simulink model "Custom_SP"  (R2020b)
settings: Solver=ode45  StartTime=0.0  StopTime=TimeScale  RelTol=1e-3
model workspace (MATLAB code in the model file):
  | %% PARAMETERS FOR CUSTOM_SP
  | %%%%%%%%%%%%%%%%%%%%% DENSITY %%%%%%%%%%%%%%%%%%%%%%%
  | al = 2.07; % g/cm^3
  | steel = 7.833; %g/cm^3
  | 
  | %%%%%%%%%%%%%%%%%%%%% BASE COORDINATES %%%%%%%%%%%%%%%%%%%%%%%
  | % Outside coordinates
  | out_base_right = [-335 -170.32; -315 -204.96;
  |     -315 -295.6; -98.49 -420.6; -20 -375.28;
  |     20 -375.28; 315 -204.96; 335 -170.32; 413.49 -125];
  | out_base_left = [413.49 125; 335 170.32;
  |     315 204.96; 20 375.28; -20 375.28;
  |     -98.49 420.6; -315 295.6; -315 204.96; -335 170.32;
  |     -335 -170.32];
  | out_base = [out_base_right; out_base_left];
  | 
  | % Inside coordinates
  | in_base = [-230 -246.52; -230 246.52; -98.49 322.45; 328.49 75.93;
  |     328.49 -75.93; -98.49 -322.45; -230 -246.52];
  | 
  | tot_base = [out_base; in_base];
  | 
  | %%%%%%%%%%%%%%%%%%%%%%% PLATE POSE ON BASE %%%%%%%%%%%%%%%%%%%%%%%%%%%
  | % PLATE POSITION ON BASE
  | plate_1 = [-272.22 -252.09 0];
  | plate_2 = [-82.21 -361.79 0];
  | plate_3 = [354.42 -109.71 0];
  | plate_4 = [354.42 109.71 0];
  | plate_5 = [-82.21 361.79 0];
  | plate_6 = [-272.22  252.09 0];
  | 
  | % ANGLE FOR JOINT ON BASE
  | plate_angle_1 = 0 + pi/2;
  | plate_angle_2 = 2*pi/3 + pi/2;
  | plate_angle_3 = 2*pi/3 + pi/2;
  | plate_angle_4 = 4*pi/3 + pi/2;
  | plate_angle_5 = 4*pi/3 + pi/2;
  | plate_angle_6 = 0 + pi/2;
  | 
  | %%%%%%%%%%%%%%%%%%%%%%%% FLANGE COORDINATES %%%%%%%%%%%%%%%%%%%%%%%%%%%%
  | flange_body = [ -20 22.5; -20 -22.5; 13.6488 -9.3106];
  | 
  | C = linspace(-68.6, 68.6, 21)';
  | C = deg2rad(C);
  | flange_round = [10+10*cos(C) 10*sin(C)];
  | 
  | C = linspace(3*pi/2, -pi/2, 100)';
  | flange_hole = [10+6*cos(C) 6*sin(C)];
  | 
  | flange = [flange_round; flange_body; flange_hole];
  | 
  | %plot(flange(:,1),flange(:,2), 'Color', [0.6 0.6 0.6], 'Marker', '.',...
  | %'MarkerSize', 9, 'MarkerEdgeColor', [1 0 0]);
  | 
  | %%%%%%%%%%%%%%%%%%%%%%%%%%%%% LID %%%%%%%%%%%%%%%%%%%%%%%%%%%%%%
  | % LID COORDINATES
  | C = linspace(-150 , -70, 9)';
  | C = deg2rad(C);
  | lid_round1 = [-171.37+10*cos(C) -103.18+10*sin(C)];
  | 
  | C = linspace(110, 60, 9)';
  | C = deg2rad(C);
  | lid_round2 = [-118.05+10*cos(C) -105.05+10*sin(C)];
  | 
  | C = linspace(60, 10, 9)';
  | C = deg2rad(C);
  | lid_round3 = [-117.46+10*cos(C) -105.39+10*sin(C)];
  | 
  | C = linspace(110, 60, 9)';
  | C = deg2rad(C);
  | lid_round4 = [-32.54+10*cos(C) -154.42+10*sin(C)];
  | 
  | C = linspace(60, 10, 9)';
  | C = deg2rad(C);
  | lid_round5 = [-31.95+10*cos(C) -154.76+10*sin(C)];
  | 
  | C = linspace(-90-80, -90, 9)';
  | C = deg2rad(C);
  | lid_round6 = [-3.67+10*cos(C) -200+10*sin(C)];
  | 
  | C = linspace(-30, 50, 9)';
  | C = deg2rad(C);
  | lid_round7 = [175.04+10*cos(C) -96.82+10*sin(C)];
  | 
  | C = linspace(-140, -90, 9)';
  | C = deg2rad(C);
  | lid_round8 = [150+10*sin(C) -49.71+10*cos(C)];
  | 
  | C = linspace(-90, -40, 9)';
  | C = deg2rad(C);
  | lid_round9 = [150+10*sin(C) -49.03+10*cos(C)];
  | 
  | C = linspace(-140, -90, 9)';
  | C = deg2rad(C);
  | lid_round10 = [150+10*sin(C) 49.03+10*cos(C)];
  | 
  | C = linspace(-90, -40, 9)';
  | C = deg2rad(C);
  | lid_round11 = [150+10*sin(C) 49.71+10*cos(C)];
  | 
  | C = linspace(-50, 30, 9)';
  | C = deg2rad(C);
  | lid_round12 = [175.04+10*cos(C) 96.82+10*sin(C)];
  | 
  | C = linspace(90, 90+80, 9)';
  | C = deg2rad(C);
  | lid_round13 = [-3.67+10*cos(C) 200+10*sin(C)];
  | 
  | C = linspace(-10, -60, 9)';
  | C = deg2rad(C);
  | lid_round14 = [-31.95+10*cos(C) 154.76+10*sin(C)];
  | 
  | C = linspace(-60, -110, 9)';
  | C = deg2rad(C);
  | lid_round15 = [-32.54+10*cos(C) 154.42+10*sin(C)];
  | 
  | C = linspace(-10, -60, 9)';
  | C = deg2rad(C);
  | lid_round16 = [-117.46+10*cos(C) 105.39+10*sin(C)];
  | 
  | C = linspace(-60, -110, 9)';
  | C = deg2rad(C);
  | lid_round17 = [-118.05+10*cos(C) 105.05+10*sin(C)];
  | 
  | C = linspace(70 , 150, 9)';
  | C = deg2rad(C);
  | lid_round18 = [-171.37+10*cos(C) 103.18+10*sin(C)];
  | 
  | lid = [-200 -73.59; lid_round1; lid_round2;
  |     lid_round3;
  |     -100.49 -144.05; -74.51 -159.05; lid_round4;
  |     lid_round5; lid_round6; 36.27 -210; 163.73 -136.41;
  |     lid_round7; lid_round8; lid_round9; 175 -15; 175 15;
  |     lid_round10; lid_round11; lid_round12; 163.73 136.41;
  |     36.27 210; lid_round13; lid_round14; lid_round15;
  |     -74.51 159.05; -100.49 144.05; lid_round16;
  |     lid_round17; lid_round18; -200 73.59];
  | 
  | lid = [-200 -73.59; lid_round1; lid_round2; lid_round3;
  |     -100.49 -144.05; -74.51 -159.05;
  |     lid_round4; lid_round5; lid_round6;
  |     36.27 -210; 163.73 -136.41;
  |     lid_round7; lid_round8; lid_round9;
  |     175 -15; 175 15;
  |     lid_round10; lid_round11; lid_round12;
  |     163.73 136.41; 36.27 210;
  |     lid_round13; lid_round14; lid_round15;
  |     -74.51 159.05; -100.49 144.05;
  |     lid_round16; lid_round17; lid_round18; -200 73.59];
  | 
  | % LID CONNECTOR
  | C = linspace(-150 , -50, 15)';
  | C = deg2rad(C);
  | lid_connector_round1 = [2.15+10*cos(C) -79.37+10*sin(C)];
  | 
  | C = linspace(-50 , 0, 15)';
  | C = deg2rad(C);
  | lid_connector_round2 = [37.5+10*cos(C) -49.71+10*sin(C)];
  | 
  | C = linspace(0 , 50, 15)';
  | C = deg2rad(C);
  | lid_connector_round3 = [37.5+10*cos(C) -49.03+10*sin(C)];
  | 
  | C = linspace(-50, 0, 15)';
  | C = deg2rad(C);
  | lid_connector_round4 = [37.5+10*cos(C) 49.03+10*sin(C)];
  | 
  | C = linspace(0, 50, 15)';
  | C = deg2rad(C);
  | lid_connector_round5 = [37.5+10*cos(C) 49.71+10*sin(C)];
  | 
  | C = linspace(50 , 150, 15)';
  | C = deg2rad(C);
  | lid_connector_round6 = [2.15+10*cos(C) 79.37+10*sin(C)];
  | 
  | lid_connector = [-12.5 -74; lid_connector_round1;
  |     lid_connector_round2; lid_connector_round3; 12.5 -15;
  |     12.5 15; lid_connector_round4; lid_connector_round5;
  |     lid_connector_round6; -12.5 74];
  | 
  | %%%%%%%%%%%%%%%%%%%%%%%%% BALL JOINT %%%%%%%%%%%%%%%%%%%%%%%%%%%
  | % BALL JOINTS
  | C = linspace(138.59, 41.41, 50)';
  | C = deg2rad(C);
  | ball_round = [10*sin(C) 10*cos(C)];
  | 
  | ball_joint = [6 -7.5; ball_round; 6 7.5];
  | 
  | % BALL CONNECTOR
  | C = linspace(-109.47, -70.53, 49)';
  | C = deg2rad(C);
  | ball_round_out = [-16*sin(C) 16*cos(C)];
  | 
  | C = linspace(-57.75, -122.25, 49)';
  | C = deg2rad(C);
  | ball_round_in = [-10*sin(C) 10*cos(C)];
  | 
  | ball_connector = [ball_round_out; ball_round_in];
  | 
  | %%%%%%%%%%%%%%%%%%%%%%%%%% MOTOR %%%%%%%%%%%%%%%%%%%%%%%%%%%
  | % KNOB UNDER MOTOR
  | C = linspace(-90+25.84, -90+64.16, 50)';
  | C = deg2rad(C);
  | knob_under_round1 = [7.5*sin(C) -7.5*cos(C)];
  | 
  | C = linspace( -64.16, -25.84, 50)';
  | C = deg2rad(C);
  | knob_under_round2 = [7.5*cos(C) 7.5*sin(C)];
  | 
  | C = linspace( 25.84, 64.16, 50)';
  | C = deg2rad(C);
  | knob_under_round3 = [7.5*cos(C) 7.5*sin(C)];
  | 
  | C = linspace( 64.16, 25.84, 50)';
  | C = deg2rad(C);
  | knob_under_round4 = [-7.5*cos(C) 7.5*sin(C)];
  | 
  | knob_under = [knob_under_round1; knob_under_round2;
  |     knob_under_round3; knob_under_round4];
  | 
  | % MOTOR UNDER
  | C = linspace(-90, -49, 10)';
  | C = deg2rad(C);
  | knob_under_round1 = [-(19+17)+5.5*sin(C) -11.13-5.5*cos(C)];
  | 
  | C = linspace(-49, 0, 10)';
  | C = deg2rad(C);
  | knob_under_round2 = [-(17+14.77)+5.5*sin(C) -16-5.5*cos(C)];
  | 
  | C = linspace(0, 180, 49)';
  | C = deg2rad(C);
  | knob_under_round3 = [20+21.5*sin(C) -21.5*cos(C)];
  | 
  | C = linspace(180, 180+49, 10)';
  | C = deg2rad(C);
  | knob_under_round4 = [-(17+14.77)+5.5*sin(C) 16-5.5*cos(C)];
  | 
  | C = linspace(270-49, 270, 10)';
  | C = deg2rad(C);
  | knob_under_round5 = [-(19+17)+5.5*sin(C) 11.13-5.5*cos(C)];
  | 
  | motor_under = [knob_under_round1; knob_under_round2;
  |     knob_under_round3; knob_under_round4; knob_under_round5];
  | 
  | % MOTOR LINEAR
  | C = linspace(-180, -101.99, 10)';
  | C = deg2rad(C);
  | motor_top_round1 = [-15.28+3*cos(C) -8.62+3*sin(C)];
  | 
  | C = linspace(-101.99, 101.99, 49)';
  | C = deg2rad(C);
  | motor_top_round2 = [3.12+15.25*cos(C) 15.25*sin(C)];
  | 
  | C = linspace(101.99, 180, 10)';
  | C = deg2rad(C);
  | motor_top_round3 = [-15.28+3*cos(C) 8.62+3*sin(C)];
  | 
  | C = linspace(180, -180, 50)';
  | C = deg2rad(C);
  | motor_top_hole = [3.12+10.1*cos(C) 10.1*sin(C)];
  | 
  | motor_linear = [motor_top_round1; motor_top_round2; motor_top_round3;
  |     -15.28-3 -8.62; motor_top_hole];
  | 
  | %%%%%%%%%%%%%%%%%%%%% MALE %%%%%%%%%%%%%%%%%%%%%%%%%%%
  | male = [15.1 -16; 15.1 16; 10.1 16;
  |     10.1 -11; 6 -11; 6 -16];
  | 
  | %%%%%%%%%%%%%%%%%%%%% FEMALE %%%%%%%%%%%%%%%%%%%%%%%%%
  | female = [15 -19; 15 19; 9.5 19; 9.5 1;
  |     5.055 1; 5.055 -19];
  | 
  | %%%%%%%%%%%%%%%%%%%%% STRAIN GAUGE %%%%%%%%%%%%%%%%%%%%%%
  | strain_gauge = [-38.1 -25.4; -22.4 -25.4; -22.4 11.6;
  |     -13.9 11.6; -13.9 -25.4; 38.1 -25.4; 38.1 25.4;
  |     22.4 25.4; 22.4 -11.6; 13.9 -11.6;
  |     13.9 25.4; -38.1 25.4];
  | 
  | %%%%%%%%%%%%%%%%%%%%% M12 STUFF %%%%%%%%%%%%%%%%%%%%%%%%%%%
  | % M12 BOLT
  | m12_bolt = [0 -18.5; 6 -18.5; 6 11.5; 10.1 11.5; 10.1 18.5; 0 18.5];
  | 
  | % M12 NUT
  | C = linspace(3*pi, pi, 50)';
  | m12_hole = [6*cos(C) 6*sin(C)];
  | m12_nut = [-21.2/2 0; -5.48 -9.5; 5.48 -9.5; 21.2/2 0; 5.48 9.5; -5.48 9.5; -21.2/2 0; m12_hole];
  | 
  | % M12 WASHER
  | m12_washer = [6 -1; 23.5/2 -1; 23.5/2 1; 6 1];
  | 
  | %%%%%%%%%%%%%%%%%%%%%% PLATFORM COORDINATES %%%%%%%%%%%%%%%%%%%%%%%%%%%
  | % Outside coordinates
  | out_platform = [36.27 -210; 163.73 -136.41;
  |     200 -73.59; 200 73.59; 163.73 136.41;
  |     36.27 210; -36.27 210; -163.73 136.41;
  |     -200 73.59; -200 -73.54; -163.73 -136.41; -36.27 -210;
  |     36.27 -210];
  | C = linspace(3*pi/2, -pi/2, 100)';
  | platform_hole = [140*cos(C) 140*sin(C)];
  | platform = [out_platform; platform_hole];
  | 
  | %%%%%%%%%%%%%%%%%%%% STUMP %%%%%%%%%%%%%%%%%%%%%%%
  | C = linspace(-pi/2, -deg2rad(12.47), 100)';
  | stump_round = [70*cos(C) -100+70*sin(C)];
  | stump = [stump_round; 100 170; 0 170];
  | 
  | %% POSITION OF BASE JOINT AND PLATFORM JOINT FOR INVERSE KINEMATICS
  | % BASE JOINT POSITION
  | plate_1;
  | plate_2;
  | plate_3;
  | plate_4;
  | plate_5;
  | plate_6;
  | 
  | zb = 35+5;
  | B = [plate_1 zb; plate_2 zb; plate_3 zb; plate_4 zb; plate_5 zb; plate_6 zb]';
  | 
  | 
  | % JOINT POSITION ON PLATFORM
  | Rot = [cos(deg2rad(120)) -sin(deg2rad(120)); sin(deg2rad(120)) cos(deg2rad(120))];
  | platform_joint_1 = [-200.54 -48.83]';
  | platform_joint_6 = [-200.54 48.83]';
  | platform_joint_2 = Rot*platform_joint_6;
  | platform_joint_3 = Rot*platform_joint_1;
  | platform_joint_4 = Rot*platform_joint_2;
  | platform_joint_5 = Rot*platform_joint_3;
  | 
  | % LEG LENGHT AT HOME POSITION
  | %ball_joint_bottom_length = 13.75; %mm
  | %nut_washer = 10 + 2 + 7.75; %mm
  | %female_length = 38 + 2; %mm
  | %motor_length = 58.5 + 163.5; %mm
  | %extender_length = 20 + 50; %mm
  | %male_bolt_nut = 5 + 7 + 25; %mm
  | %strain_gauge_length = 38.1*2; %mm
  | %nut = 10 + 7.75; %mm
  | %ball_joint_top_length = 13.75; %mm
  | 
  | %leg_initial_length = ball_joint_bottom_length + nut_washer + female_length + motor_length + extender_length + male_bolt_nut + strain_gauge_length + nut + ball_joint_top_length;
  | 
  | %leg_initial_length = 510.2061739;
  | 
  | %height_home = sqrt(leg_initial_length^2 - (plate_1(1)-platform_joint_1(1))^2 - (plate_1(2)-platform_joint_1(2))^2) + zb;
  | height_home = 503.318 + 2.5;
  | P = [platform_joint_1' height_home; platform_joint_2' height_home; platform_joint_3' height_home; platform_joint_4' height_home; platform_joint_5' height_home; platform_joint_6' height_home]';
values from neighbouring files (symbols this model uses):
  LegSpring = 50000    [SP_parameters.m]
undefined symbols (not defined in the file or in its folder): X, Y, Z
libraries: nesl_utility x13, Custom_SP_lib x8, sm_lib x7, simulink x6
settings Model: Creator=ellen  LastModifiedBy=axelzedigh

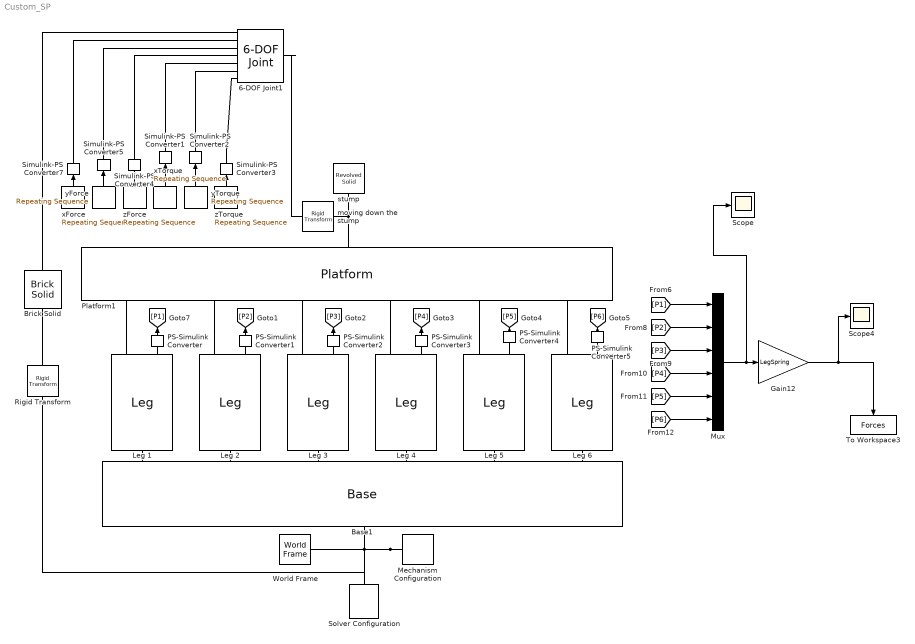
== system Custom_SP ==
  6-DOF Joint1 : sm_lib/Joints/6-DOF Joint  JointMode=Normal  SenseConstraintForce=off  SenseConstraintForceX=off  SenseConstraintForceY=off  SenseConstraintForceZ=off  SenseConstraintTorque=off  SenseConstraintTorqueX=off  SenseConstraintTorqueY=off  SenseConstraintTorqueZ=off  SenseTotalForce=off  SenseTotalForceX=off  SenseTotalForceY=off  SenseTotalForceZ=off  SenseTotalTorque=off  SenseTotalTorqueX=off  SenseTotalTorqueY=off  SenseTotalTorqueZ=off  CompositeWrenchDir=FollowerOnBase  CompositeWrenchFrame=BaseFrame  PxEquilibriumPosition=0  PxEquilibriumPositionUnits=m  PxSpringStiffness=0  PxSpringStiffnessUnits=N/m  PxDampingCoefficient=0  PxDampingCoefficientUnits=N/(m/s)  PxTorqueActuationMode=InputTorque  PxMotionActuationMode=ComputedMotion  PxSensePosition=off  PxSenseVelocity=off  PxSenseAcceleration=off  PxSenseTorqueForce=off  PxSenseLowerLimitTorqueForce=off  PxSenseUpperLimitTorqueForce=off  PxLowerLimitSpecify=off  PxLowerLimitBound=-1  PxLowerLimitBoundUnits=m  PxLowerLimitStiffness=1e6  PxLowerLimitStiffnessUnits=N/m  PxLowerLimitDamping=1e3  PxLowerLimitDampingUnits=N/(m/s)  PxLowerLimitTransitionRegionWidth=1e-4  PxLowerLimitTransitionRegionWidthUnits=m  PxUpperLimitSpecify=off  PxUpperLimitBound=1  PxUpperLimitBoundUnits=m  PxUpperLimitStiffness=1e6  PxUpperLimitStiffnessUnits=N/m  PxUpperLimitDamping=1e3  PxUpperLimitDampingUnits=N/(m/s)  PxUpperLimitTransitionRegionWidth=1e-4  PxUpperLimitTransitionRegionWidthUnits=m  PxPositionTargetSpecify=off  PxPositionTargetPriority=High  PxPositionTargetValue=0  PxPositionTargetValueUnits=m  PxVelocityTargetSpecify=off  PxVelocityTargetPriority=High  PxVelocityTargetValue=0  PxVelocityTargetValueUnits=m/s  PyEquilibriumPosition=0  PyEquilibriumPositionUnits=m  PySpringStiffness=0  PySpringStiffnessUnits=N/m  PyDampingCoefficient=0  PyDampingCoefficientUnits=N/(m/s)  PyTorqueActuationMode=InputTorque  PyMotionActuationMode=ComputedMotion  PySensePosition=off  PySenseVelocity=off  PySenseAcceleration=off  PySenseTorqueForce=off  PySenseLowerLimitTorqueForce=off  PySenseUpperLimitTorqueForce=off  PyLowerLimitSpecify=off  PyLowerLimitBound=-1  PyLowerLimitBoundUnits=m  PyLowerLimitStiffness=1e6  PyLowerLimitStiffnessUnits=N/m  PyLowerLimitDamping=1e3  PyLowerLimitDampingUnits=N/(m/s)  PyLowerLimitTransitionRegionWidth=1e-4  PyLowerLimitTransitionRegionWidthUnits=m  PyUpperLimitSpecify=off  PyUpperLimitBound=1  PyUpperLimitBoundUnits=m  PyUpperLimitStiffness=1e6  PyUpperLimitStiffnessUnits=N/m  PyUpperLimitDamping=1e3  PyUpperLimitDampingUnits=N/(m/s)  PyUpperLimitTransitionRegionWidth=1e-4  PyUpperLimitTransitionRegionWidthUnits=m  PyPositionTargetSpecify=off  PyPositionTargetPriority=High  PyPositionTargetValue=0  PyPositionTargetValueUnits=m  PyVelocityTargetSpecify=off  PyVelocityTargetPriority=High  PyVelocityTargetValue=0  PyVelocityTargetValueUnits=m/s  PzEquilibriumPosition=0  PzEquilibriumPositionUnits=m  PzSpringStiffness=0  PzSpringStiffnessUnits=N/m  PzDampingCoefficient=0  PzDampingCoefficientUnits=N/(m/s)  PzTorqueActuationMode=InputTorque  PzMotionActuationMode=ComputedMotion  PzSensePosition=off  PzSenseVelocity=off  PzSenseAcceleration=off  PzSenseTorqueForce=off  PzSenseLowerLimitTorqueForce=off  PzSenseUpperLimitTorqueForce=off  PzLowerLimitSpecify=off  PzLowerLimitBound=-1  PzLowerLimitBoundUnits=m  PzLowerLimitStiffness=1e6  PzLowerLimitStiffnessUnits=N/m  PzLowerLimitDamping=1e3  PzLowerLimitDampingUnits=N/(m/s)  PzLowerLimitTransitionRegionWidth=1e-4  PzLowerLimitTransitionRegionWidthUnits=m  PzUpperLimitSpecify=off  PzUpperLimitBound=1  PzUpperLimitBoundUnits=m  PzUpperLimitStiffness=1e6  PzUpperLimitStiffnessUnits=N/m  PzUpperLimitDamping=1e3  PzUpperLimitDampingUnits=N/(m/s)  PzUpperLimitTransitionRegionWidth=1e-4  PzUpperLimitTransitionRegionWidthUnits=m  PzPositionTargetSpecify=off  PzPositionTargetPriority=High  PzPositionTargetValue=0  PzPositionTargetValueUnits=m  PzVelocityTargetSpecify=off  PzVelocityTargetPriority=High  PzVelocityTargetValue=0  PzVelocityTargetValueUnits=m/s  SphDefPosRotationMethod=None  SphDefPosRotationAngleUnits=deg  SphDefPosRotationStandardAxis=+Z  SphDefPosRotationAngle=0.0  SphDefPosRotationArbitraryAxis=[0 0 1]  SphDefPosFollAlignAxisA=+X  SphDefPosBaseAlignAxisA=+Y  SphDefPosFollAlignAxisB=+Y  SphDefPosBaseAlignAxisB=+Z  SphDefPosRotationSequenceAxes=FollowerAxes  SphDefPosRotationSequence=XYX  SphDefPosRotationSequenceAngles=[0 0 0]  SphDefPosRotationSequenceAnglesUnits=deg  SphDefPosRotationMatrix=[1 0 0; 0 1 0; 0 0 1]  SphEqPosRotationMethod=None  SphEqPosRotationAngleUnits=deg  SphEqPosRotationStandardAxis=+Z  SphEqPosRotationAngle=0.0  SphEqPosRotationArbitraryAxis=[0 0 1]  SphEqPosFollAlignAxisA=+X  SphEqPosBaseAlignAxisA=+Y  SphEqPosFollAlignAxisB=+Y  SphEqPosBaseAlignAxisB=+Z  SphEqPosRotationSequenceAxes=FollowerAxes  SphEqPosRotationSequence=XYX  SphEqPosRotationSequenceAngles=[0 0 0]  SphEqPosRotationSequenceAnglesUnits=deg  SphEqPosRotationMatrix=[1 0 0; 0 1 0; 0 0 1]  SphSpringStiffness=0  SphSpringStiffnessUnits=N*m/deg  SphDampingCoefficient=0  SphDampingCoefficientUnits=N*m/(deg/s)  SphActuateTorqueX=on  SphActuateTorqueY=on  SphActuateTorqueZ=on  SphActuateTorque=off  SphTorqueActuationMode=InputTorque  SphMotionActuationMode=ComputedMotion  SphActuationFrame=BaseFrame  SphSensePosition=off  SphSenseVelocityX=off  SphSenseVelocityY=off  SphSenseVelocityZ=off  SphSenseVelocity=off  SphSenseAccelerationX=off  SphSenseAccelerationY=off  SphSenseAccelerationZ=off  SphSenseAcceleration=off  SphSenseTorqueX=off  SphSenseTorqueY=off  SphSenseTorqueZ=off  SphSenseTorqueForce=off  SphSenseLowerLimitTorqueMag=off  SphSenseUpperLimitTorqueMag=off  SphSensingFrame=BaseFrame  SphLowerLimitSpecify=off  SphLowerLimitBound=15  SphLowerLimitBoundUnits=deg  SphLowerLimitStiffness=1e4  SphLowerLimitStiffnessUnits=N*m/deg  SphLowerLimitDamping=10  SphLowerLimitDampingUnits=N*m/(deg/s)  SphLowerLimitTransitionRegionWidth=0.1  SphLowerLimitTransitionRegionWidthUnits=deg  SphUpperLimitSpecify=off  SphUpperLimitBound=45  SphUpperLimitBoundUnits=deg  SphUpperLimitStiffness=1e4  SphUpperLimitStiffnessUnits=N*m/deg  SphUpperLimitDamping=10  SphUpperLimitDampingUnits=N*m/(deg/s)  SphUpperLimitTransitionRegionWidth=0.1  SphUpperLimitTransitionRegionWidthUnits=deg  SphPositionTargetRotationMethod=None  SphPositionTargetRotationAngleUnits=deg  SphPositionTargetRotationStandardAxis=+Z  SphPositionTargetRotationAngle=0.0  SphPositionTargetRotationArbitraryAxis=[0 0 1]  SphPositionTargetFollAlignAxisA=+X  SphPositionTargetBaseAlignAxisA=+Y  SphPositionTargetFollAlignAxisB=+Y  SphPositionTargetBaseAlignAxisB=+Z  SphPositionTargetRotationSequenceAxes=FollowerAxes  SphPositionTargetRotationSequence=XYX  SphPositionTargetRotationSequenceAngles=[0 0 0]  SphPositionTargetRotationSequenceAnglesUnits=deg  SphPositionTargetRotationMatrix=[1 0 0; 0 1 0; 0 0 1]  SphPositionTargetSpecify=off  SphPositionTargetPriority=High  SphVelocityTargetValue=[0 0 0]  SphVelocityTargetValueUnits=deg/s  SphVelocityTargetSpecify=off  SphVelocityTargetPriority=High  SphVelocityTargetInFollowerFrame=on
  Base1 : Custom_SP_lib/Base  SystemSampleTime=-1  VariantActivationTime=update diagram  Latency=0  AutoFrameSizeCalculation=off
  Brick Solid : sm_lib/Body Elements/Brick Solid  GraphicAmbientColor=[0.15 0.15 0.15 1.0]  BasedOnType=Density  BrickDimensions=[1 1 1]  BrickDimensionUnits=cm  CenterOfMass=[0 0 0]  CenterOfMassUnits=m  GraphicDiffuseColor=[0.5 0.5 0.5]  Density=1000  DensityUnits=kg/m^3  DoExposeReferenceFrame=off  GraphicEmissiveColor=[0.0 0.0 0.0 1.0]  ExportEntireGeometry=off  SerializedFrames=<Frames><Frame><Id>Frame1</Id><Value><Name>joint</Name><Origin><Source>GeometricFeature</Source><FeatureName>+z surface</FeatureName></Origin><PrimaryAxis><DefinedDirection>+Z</DefinedDirection><Source>ReferenceFrame</Source><SourceDirection>+Z</SourceDirection><FeatureName></FeatureName></PrimaryAxis><SecondaryAxis><DefinedDirection>+X</DefinedDirection><Source>ReferenceFrame</Source><SourceDirection>+X</SourceDirection><FeatureName></FeatureName></SecondaryAxis></Value></Frame><Frame><Id>Frame2</Id><Value><Name>base</Name><Origin><Source>GeometricFeature</Source><FeatureName>-z surface</FeatureName></Origin><PrimaryAxis><DefinedDirection>+Z</DefinedDirection><Source>ReferenceFrame</Source><SourceDirection>+Z</SourceDirection><FeatureName></FeatureName></PrimaryAxis><SecondaryAxis><DefinedDirection>+X</DefinedDirection><Source>ReferenceFrame</Source><SourceDirection>+X</SourceDirection><FeatureName></FeatureName></SecondaryAxis></Value></Frame></Frames>  MarkerShape=Sphere  MarkerSize=10  GraphicType=FromGeometry  InertiaType=CalculateFromGeometry  Mass=1  MassUnits=kg  MomentsOfInertia=[1 1 1]  MomentsOfInertiaUnits=kg*m^2  GraphicOpacity=1.0  ProductsOfInertia=[0 0 0]  ProductsOfInertiaUnits=kg*m^2  GraphicShininess=75  GraphicSpecularColor=[0.5 0.5 0.5 1.0]  GraphicVisPropType=SimpleVisualProperties
  Gain12 : Gain  Gain=LegSpring
  Leg {1..6} (6 alike) : Custom_SP_lib/Leg  SystemSampleTime=-1  VariantActivationTime=update diagram  Latency=0  AutoFrameSizeCalculation=off
  Mechanism Configuration : sm_lib/Utilities/Mechanism Configuration  UniformGravity=Constant  GravityVector=[0 0 -9.81]  GravityVectorUnits=m/s^2  GravityUnits=m/s^2  LinearizationDelta=0.001  JointModeTransitionNonlinearIterations=2
  Mux : Mux  Inputs=6
  PS-Simulink Converter{,1..5} (6 alike) : nesl_utility/PS-Simulink Converter  PhysicalDomain=network_engine_domain  SubClassName=ps_output  LeftPortType=input  RightPortType=output  PseudoPeriodic=off  Frequencies=[]  Unit=inherit  AffineConversion=off
  Platform1 : Custom_SP_lib/Platform  SystemSampleTime=-1  VariantActivationTime=update diagram  Latency=0  AutoFrameSizeCalculation=off
  Rigid Transform : sm_lib/Frames and Transforms/Rigid Transform  TranslationMethod=StandardAxis  TranslationStandardOffset=height_home-2.5-200-10-10  TranslationLengthUnit=mm  TranslationStandardAxis=+Z  TranslationCartesianOffset=[0 0 0]  TranslationROffset=0  TranslationROffsetUnits=m  TranslationZOffset=0  TranslationZOffsetUnits=m  TranslationThetaOffset=0  TranslationThetaOffsetUnits=deg  RotationMethod=None  RotationAngleUnits=deg  RotationStandardAxis=+Z  RotationAngle=0.0  RotationArbitraryAxis=[0 0 1]  FollAlignAxisA=+X  BaseAlignAxisA=+Y  FollAlignAxisB=+Y  BaseAlignAxisB=+Z  RotationSequenceAxes=FollowerAxes  RotationSequence=XYX  RotationSequenceAngles=[0 0 0]  RotationSequenceAnglesUnits=deg  RotationMatrix=[1 0 0; 0 1 0; 0 0 1]
  Scope : Scope
  Scope4 : Scope
  Simulink-PS Converter1 : nesl_utility/Simulink-PS Converter  PhysicalDomain=network_engine_domain  SubClassName=ps_input  LeftPortType=input  RightPortType=output  PseudoPeriodic=off  Frequencies=[]  NoiseDistribution=none  NoiseParameters=[]  Unit=N*m  AffineConversion=off  FilteringAndDerivatives=provide  SimscapeFilterOrder=1  InputFilterTimeConstant=0.001  UdotUserProvided=0
  Simulink-PS Converter2 : nesl_utility/Simulink-PS Converter  PhysicalDomain=network_engine_domain  SubClassName=ps_input  LeftPortType=input  RightPortType=output  PseudoPeriodic=off  Frequencies=[]  NoiseDistribution=none  NoiseParameters=[]  Unit=N*m  AffineConversion=off  FilteringAndDerivatives=provide  SimscapeFilterOrder=1  InputFilterTimeConstant=0.001  UdotUserProvided=0
  Simulink-PS Converter3 : nesl_utility/Simulink-PS Converter  PhysicalDomain=network_engine_domain  SubClassName=ps_input  LeftPortType=input  RightPortType=output  PseudoPeriodic=off  Frequencies=[]  NoiseDistribution=none  NoiseParameters=[]  Unit=N*m  AffineConversion=off  FilteringAndDerivatives=provide  SimscapeFilterOrder=1  InputFilterTimeConstant=0.001  UdotUserProvided=0
  Simulink-PS Converter4 : nesl_utility/Simulink-PS Converter  PhysicalDomain=network_engine_domain  SubClassName=ps_input  LeftPortType=input  RightPortType=output  PseudoPeriodic=off  Frequencies=[]  NoiseDistribution=none  NoiseParameters=[]  Unit=N  AffineConversion=off  FilteringAndDerivatives=provide  SimscapeFilterOrder=1  InputFilterTimeConstant=0.001  UdotUserProvided=0
  Simulink-PS Converter5 : nesl_utility/Simulink-PS Converter  PhysicalDomain=network_engine_domain  SubClassName=ps_input  LeftPortType=input  RightPortType=output  PseudoPeriodic=off  Frequencies=[]  NoiseDistribution=none  NoiseParameters=[]  Unit=N  AffineConversion=off  FilteringAndDerivatives=provide  SimscapeFilterOrder=1  InputFilterTimeConstant=0.001  UdotUserProvided=0
  Simulink-PS Converter7 : nesl_utility/Simulink-PS Converter  PhysicalDomain=network_engine_domain  SubClassName=ps_input  LeftPortType=input  RightPortType=output  PseudoPeriodic=off  Frequencies=[]  NoiseDistribution=none  NoiseParameters=[]  Unit=N  AffineConversion=off  FilteringAndDerivatives=provide  SimscapeFilterOrder=1  InputFilterTimeConstant=0.001  UdotUserProvided=0
  Solver Configuration : nesl_utility/Solver Configuration  PhysicalDomain=network_engine_domain  SubClassName=solver  LeftPortType=input  RightPortType=generic  Tones=[]  Harmonics=[]  SimulateNoise=off  Profile=off  UseLocalSampling=off  EnableSwitchedLinearOptims=on  FrequencyDomain=off  UseCCode=off  RelTol=0.001  AbsTol=1e-06  MinStep=1e-09  ToWorkspace=off  RevertToSquareIcSolve=off  NumHomotopyIterations=100  PhasorMode=off  PhasorModeNumHarmonics=1  DoDC=off  ResidualTolerance=1e-9  UseLocalSolver=off  LocalSolverChoice=NE_BACKWARD_EULER_ADVANCER  LocalSolverSampleTime=.001  DoFixedCost=off  MaxNonlinIter=3  MaxModeIter=2  ComputeImpulses=off  ImpulseIterations=2  LinearAlgebra=Sparse  EquationFormulation=NE_TIME_EF  DelaysMemoryBudget=1024  AutomaticFiltering=on  FilteringTimeConstant=0.001  PartitionStorageMethod=AS_NEEDED  PartitionMemoryBudget=1024  PartitionMethod=FAST
  To Workspace3 : ToWorkspace  VariableName=Forces  SaveFormat=Structure With Time  SampleTime=-1
  World Frame : sm_lib/Frames and Transforms/World Frame
  moving down the stump : sm_lib/Frames and Transforms/Rigid Transform  TranslationMethod=StandardAxis  TranslationStandardOffset=20  TranslationLengthUnit=cm  TranslationStandardAxis=+Z  TranslationCartesianOffset=[0 0 0]  TranslationROffset=0  TranslationROffsetUnits=m  TranslationZOffset=0  TranslationZOffsetUnits=m  TranslationThetaOffset=0  TranslationThetaOffsetUnits=deg  RotationMethod=AlignedAxes  RotationAngleUnits=deg  RotationStandardAxis=+Y  RotationAngle=90  RotationArbitraryAxis=[0 0 1]  FollAlignAxisA=+Z  BaseAlignAxisA=+Z  FollAlignAxisB=+X  BaseAlignAxisB=-X  RotationSequenceAxes=FollowerAxes  RotationSequence=XYX  RotationSequenceAngles=[0 0 0]  RotationSequenceAnglesUnits=deg  RotationMatrix=[1 0 0; 0 1 0; 0 0 1]
      settings: SourceProductName=Multibody
  stump : sm_lib/Body Elements/Revolved Solid  GraphicAmbientColor=[0.15 0.15 0.15 1.0]  BasedOnType=Density  CenterOfMass=[0 0 0]  CenterOfMassUnits=m  GraphicDiffuseColor=2*[0.5 0.5 0.5]  ExportConvexHullGeometry=off  Density=1000  DensityUnits=kg/m^3  DoExposeReferenceFrame=off  GraphicEmissiveColor=[0.0 0.0 0.0 1.0]  ExportEntireGeometry=off  SerializedFrames=<Frames><Frame><Id>Frame1</Id><Value><Name>top</Name><Origin><Source>GeometricFeature</Source><FeatureName>side surface 3</FeatureName></Origin><PrimaryAxis><DefinedDirection>+Z</DefinedDirection><Source>ReferenceFrame</Source><SourceDirection>+Z</SourceDirection><FeatureName></FeatureName></PrimaryAxis><SecondaryAxis><DefinedDirection>+X</DefinedDirection><Source>ReferenceFrame</Source><SourceDirection>+X</SourceDirection><FeatureName></FeatureName></SecondaryAxis></Value></Frame></Frames>  MarkerShape=Sphere  MarkerSize=10  GraphicType=FromGeometry  InertiaType=CalculateFromGeometry  Mass=1  MassUnits=kg  MomentsOfInertia=[1 1 1]  MomentsOfInertiaUnits=kg*m^2  GraphicOpacity=1.0  ProductsOfInertia=[0 0 0]  ProductsOfInertiaUnits=kg*m^2  RevolutionCrossSection=stump  RevolutionCrossSectionUnits=mm  RevolutionAngle=180  RevolutionAngleUnits=deg  RevolutionExtent=Full  GraphicShininess=75  GraphicSpecularColor=[0.5 0.5 0.5 1.0]  GraphicVisPropType=SimpleVisualProperties
  xForce : simulink/Sources/Repeating Sequence  rep_seq_t=TIME  rep_seq_y=FX
  xTorque : simulink/Sources/Repeating Sequence  rep_seq_t=TIME  rep_seq_y=MX
  yForce : simulink/Sources/Repeating Sequence  rep_seq_t=TIME  rep_seq_y=FY
  yTorque : simulink/Sources/Repeating Sequence  rep_seq_t=TIME  rep_seq_y=MY
  zForce : simulink/Sources/Repeating Sequence  rep_seq_t=TIME  rep_seq_y=FZ
  zTorque : simulink/Sources/Repeating Sequence  rep_seq_t=TIME  rep_seq_y=MZ
  wires:
  PS-Simulink Converter/1 -> [P1]
  PS-Simulink Converter1/1 -> [P2]
  PS-Simulink Converter2/1 -> [P3]
  PS-Simulink Converter3/1 -> [P4]
  PS-Simulink Converter5/1 -> [P6]
  [P5] -> Mux/5
  [P2] -> Mux/2
  [P3] -> Mux/3
  [P1] -> Mux/1
  [P4] -> Mux/4
  [P6] -> Mux/6
  zTorque/1 -> Simulink-PS Converter3/1
  xTorque/1 -> Simulink-PS Converter1/1
  zForce/1 -> Simulink-PS Converter4/1
  xForce/1 -> Simulink-PS Converter7/1
  Gain12/1 -> To Workspace3/1, Scope4/1
  Mux/1 -> Scope/1, Gain12/1
  PS-Simulink Converter4/1 -> [P5]
  yForce/1 -> Simulink-PS Converter5/1
  yTorque/1 -> Simulink-PS Converter2/1
  connections:
  Leg 1/RConn1 -- Platform1/RConn1
  Leg 1/LConn1 -- Base1/LConn1
  Leg 2/LConn1 -- Base1/LConn2
  Leg 3/LConn1 -- Base1/LConn3
  Leg 4/LConn1 -- Base1/LConn4
  Leg 5/LConn1 -- Base1/LConn5
  Leg 6/LConn1 -- Base1/LConn6
  Leg 1/RConn2 -- PS-Simulink Converter/LConn1
  Leg 2/RConn2 -- PS-Simulink Converter1/LConn1
  Leg 3/RConn2 -- PS-Simulink Converter2/LConn1
  Leg 4/RConn2 -- PS-Simulink Converter3/LConn1
  Leg 5/RConn2 -- PS-Simulink Converter4/LConn1
  Leg 6/RConn2 -- PS-Simulink Converter5/LConn1
  Mechanism Configuration/RConn1 -- Rigid Transform/LConn1 -- Solver Configuration/RConn1 -- Base1/RConn1 -- World Frame/RConn1
  Leg 2/RConn1 -- Platform1/RConn2
  Leg 3/RConn1 -- Platform1/RConn3
  Leg 4/RConn1 -- Platform1/RConn4
  Leg 5/RConn1 -- Platform1/RConn5
  Leg 6/RConn1 -- Platform1/RConn6
  moving down the stump/RConn1 -- stump/LConn1 -- Platform1/LConn1
  Rigid Transform/RConn1 -- Brick Solid/RConn1
  Brick Solid/LConn1 -- 6-DOF Joint1/LConn1
  6-DOF Joint1/RConn1 -- moving down the stump/LConn1
  Simulink-PS Converter7/RConn1 -- 6-DOF Joint1/LConn2
  Simulink-PS Converter5/RConn1 -- 6-DOF Joint1/LConn3
  Simulink-PS Converter4/RConn1 -- 6-DOF Joint1/LConn4
  Simulink-PS Converter1/RConn1 -- 6-DOF Joint1/LConn5
  Simulink-PS Converter2/RConn1 -- 6-DOF Joint1/LConn6
  Simulink-PS Converter3/RConn1 -- 6-DOF Joint1/LConn7
